simulink model "untitled"  (R2012b)
settings: Solver=ode3  StartTime=0.0  StopTime=3.5  FixedStep=1e-5/2  RelTol=1e-6
libraries: simulink x3
settings Model: Creator=Juliano  LastModifiedBy=Juliano

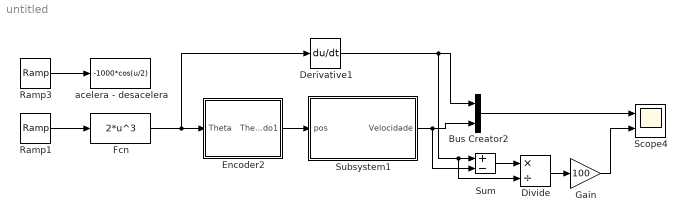
== system untitled ==
  Bus Creator2 : BusCreator  Inputs=2
  Derivative1 : Derivative
  Divide : Product  Inputs=*/
  Encoder2 : Subsystem  mask{Nr=300}
      mask prompts: Nr "Número de pulsos por revolução"
  Fcn : Fcn  Expr=2*u^3
  Gain : Gain  Gain=100
  Ramp1 : simulink/Sources/Ramp  slope=10  start=0  X0=0
  Ramp3 : simulink/Sources/Ramp  slope=2*pi  start=0  X0=0
  Scope4 : Scope  NumInputPorts=2
      settings: TickLabels=on  YMin=0~-30  YMax=30~30  SaveName=ScopeData4
  Subsystem1 : Subsystem  mask{Ts=0.01}
      mask prompts: Ts "Sampling time"
  Sum : Sum  Inputs=+-
  acelera - desacelera : Fcn  Expr=-1000*cos(u/2)
  wires:
  Ramp1/1 -> Fcn/1
  Fcn/1 -> Derivative1/1, Encoder2/1(Theta)
  Bus Creator2/1 -> Scope4/1
  Encoder2/1(Theta_amostrado1) -> Subsystem1/1(pos)
  Subsystem1/1(Velocidade) -> Sum/2, Bus Creator2/2
  Derivative1/1 -> Divide/2, Sum/1, Bus Creator2/1
  Sum/1 -> Divide/1
  Divide/1 -> Gain/1
  Gain/1 -> Scope4/2
  Ramp3/1 -> acelera - desacelera/1

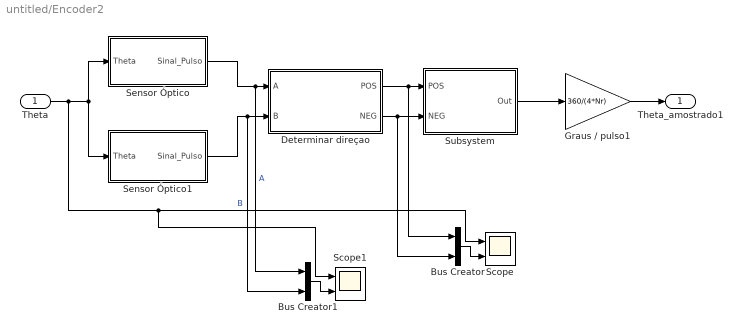
== system untitled/Encoder2 ==
  Theta : Inport
  Bus Creator : BusCreator  Inputs=2
  Bus Creator1 : BusCreator  Inputs=2
  Determinar direçao : Subsystem
  Graus / pulso1 : Gain  Gain=360/(4*Nr)  OutDataTypeStr=double
  Scope : Scope  NumInputPorts=2
      settings: YMin=-1~-5  YMax=1.5~5  SaveName=ScopeData5
  Scope1 : Scope  NumInputPorts=2
      settings: YMin=-1~-5  YMax=1.5~5  SaveName=ScopeData6
  Sensor Óptico : Subsystem
  Sensor Óptico1 : Subsystem
  Subsystem : Subsystem
  Theta_amostrado1 : Outport
  wires:
  Sensor Óptico/1(Sinal_Pulso) -> Bus Creator1/1, Determinar direçao/1(A)  "A"
  Sensor Óptico1/1(Sinal_Pulso) -> Bus Creator1/2, Determinar direçao/2(B)  "B"
  Determinar direçao/1(POS) -> Bus Creator/1, Subsystem/1(POS)
  Determinar direçao/2(NEG) -> Bus Creator/2, Subsystem/2(NEG)
  Subsystem/1(Out) -> Graus / pulso1/1
  Graus / pulso1/1 -> Theta_amostrado1/1
  Bus Creator/1 -> Scope/2
  Theta/1 -> Scope1/1, Scope/1, Sensor Óptico1/1(Theta), Sensor Óptico/1(Theta)
  Bus Creator1/1 -> Scope1/2

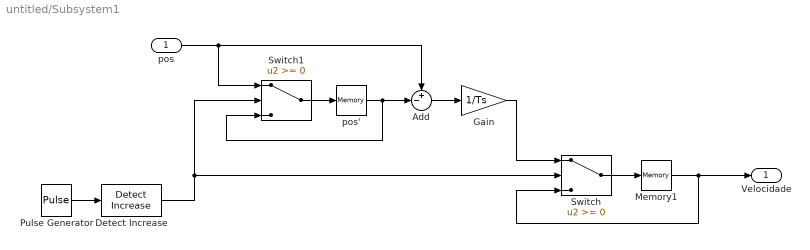
== system untitled/Subsystem1 ==
  pos : Inport
  Add : Sum  Inputs=+-|
  Detect Increase : simulink/Logic and Bit Operations/Detect Increase  vinit=0.0  InputProcessing=Inherited  OutDataTypeStr=boolean
  Gain : Gain  Gain=1/Ts
  Memory1 : Memory
  Pulse Generator : DiscretePulseGenerator  PulseType=Time based  Period=Ts  PulseWidth=50
  Switch : Switch
  Switch1 : Switch
  pos' : Memory
  Velocidade : Outport
  wires:
  pos'/1 -> Add/2, Switch1/3
  Pulse Generator/1 -> Detect Increase/1
  Add/1 -> Gain/1
  Switch1/1 -> pos'/1
  Switch/1 -> Memory1/1
  Memory1/1 -> Velocidade/1, Switch/3
  pos/1 -> Switch1/1, Add/1
  Gain/1 -> Switch/1
  Detect Increase/1 -> Switch/2, Switch1/2

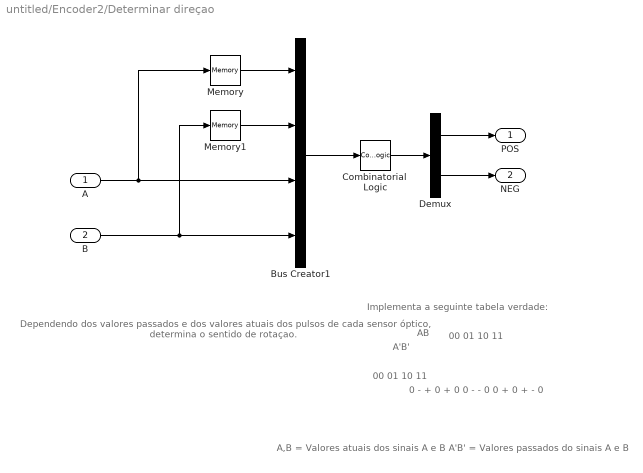
== system untitled/Encoder2/Determinar direçao ==
  note: A,B = Valores atuais dos sinais A e B
      | A'B' = Valores passados do sinais A e B
  note: A'B'
  note: AB
  note: Implementa a seguinte tabela verdade:
  note: 0	-	+	0
      | +	0	0	-
      | -	0	0	+
      | 0	+	-	0
  note: 00 01 10 11
  note: 00
      | 01
      | 10
      | 11
  note: Dependendo dos valores passados e dos valores atuais
      | dos pulsos de cada sensor óptico, determina o sentido
      | de rotaçao.
  A : Inport
  B : Inport  Port=2
  Bus Creator1 : BusCreator
  Combinatorial  Logic : CombinatorialLogic  TruthTable=[ 0 0 ; 0 1 ; 1 0 ; 0 0 ; 1 0 ; 0 0 ; 0 0 ; 0 1 ; 0 1 ; 0 0 ; 0 0 ; 1 0 ; 0 0 ; 1 0 ; 0 1 ; 0 0]
  Demux : Demux  Outputs=2
  Memory : Memory
  Memory1 : Memory
  POS : Outport
  NEG : Outport  Port=2
  wires:
  Demux/1 -> POS/1
  A/1 -> Memory/1, Bus Creator1/3
  Demux/2 -> NEG/1
  Combinatorial  Logic/1 -> Demux/1
  Memory/1 -> Bus Creator1/1
  Bus Creator1/1 -> Combinatorial  Logic/1
  Memory1/1 -> Bus Creator1/2
  B/1 -> Memory1/1, Bus Creator1/4

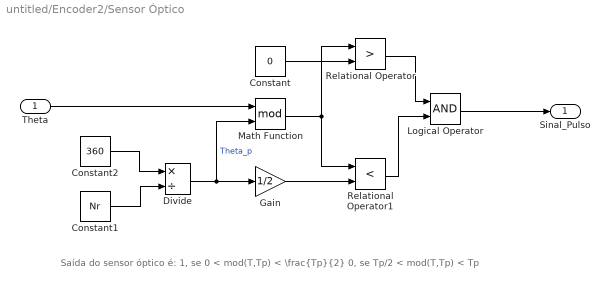
== system untitled/Encoder2/Sensor Óptico ==
  note: Saída do sensor óptico é:
      | 1, se	0 < mod(T,Tp) < \frac{Tp}{2}
      |  0, se      Tp/2 < mod(T,Tp) < Tp
  Theta : Inport
  Constant : Constant  Value=0
  Constant1 : Constant  Value=Nr
  Constant2 : Constant  Value=360
  Divide : Product  Inputs=*/
  Gain : Gain  Gain=1/2
  Logical Operator : Logic  AllPortsSameDT=off  OutDataTypeStr=boolean
  Math Function : Math  Operator=mod  SaturateOnIntegerOverflow=on
  Relational Operator : RelationalOperator  Operator=>  OutDataTypeStr=boolean
  Relational Operator1 : RelationalOperator  Operator=<  OutDataTypeStr=boolean
  Sinal_Pulso : Outport
  wires:
  Math Function/1 -> Relational Operator1/1, Relational Operator/1
  Theta/1 -> Math Function/1
  Relational Operator/1 -> Logical Operator/1
  Relational Operator1/1 -> Logical Operator/2
  Constant/1 -> Relational Operator/2
  Divide/1 -> Math Function/2, Gain/1  "Theta_p"
  Gain/1 -> Relational Operator1/2
  Logical Operator/1 -> Sinal_Pulso/1
  Constant2/1 -> Divide/1
  Constant1/1 -> Divide/2

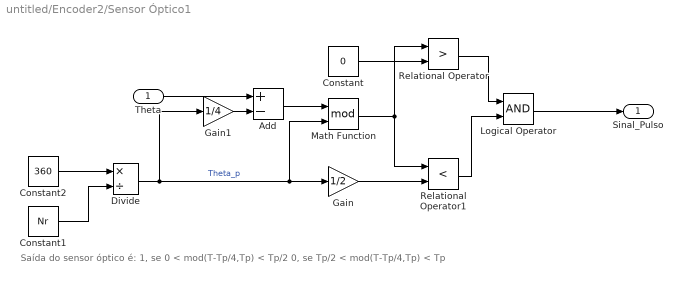
== system untitled/Encoder2/Sensor Óptico1 ==
  note: Saída do sensor óptico é:
      | 1, se	0 < mod(T-Tp/4,Tp) < Tp/2
      |  0, se     Tp/2 < mod(T-Tp/4,Tp) < Tp
  Theta : Inport
  Add : Sum  Inputs=+-
  Constant : Constant  Value=0
  Constant1 : Constant  Value=Nr
  Constant2 : Constant  Value=360
  Divide : Product  Inputs=*/
  Gain : Gain  Gain=1/2
  Gain1 : Gain  Gain=1/4
  Logical Operator : Logic  AllPortsSameDT=off  OutDataTypeStr=boolean
  Math Function : Math  Operator=mod  SaturateOnIntegerOverflow=on
  Relational Operator : RelationalOperator  Operator=>  OutDataTypeStr=boolean
  Relational Operator1 : RelationalOperator  Operator=<  OutDataTypeStr=boolean
  Sinal_Pulso : Outport
  wires:
  Constant1/1 -> Divide/2
  Constant2/1 -> Divide/1
  Logical Operator/1 -> Sinal_Pulso/1
  Gain/1 -> Relational Operator1/2
  Divide/1 -> Gain1/1, Gain/1, Math Function/2  "Theta_p"
  Constant/1 -> Relational Operator/2
  Relational Operator1/1 -> Logical Operator/2
  Relational Operator/1 -> Logical Operator/1
  Math Function/1 -> Relational Operator/1, Relational Operator1/1
  Add/1 -> Math Function/1
  Theta/1 -> Add/1
  Gain1/1 -> Add/2

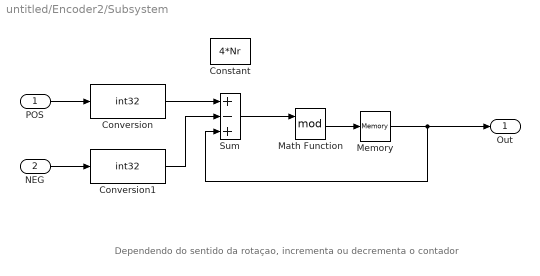
== system untitled/Encoder2/Subsystem ==
  note: Dependendo do sentido da rotaçao, incrementa ou decrementa o contador
  POS : Inport
  NEG : Inport  Port=2
  Constant : Constant  Value=4*Nr
  Conversion : DataTypeConversion  OutDataTypeStr=int32
  Conversion1 : DataTypeConversion  OutDataTypeStr=int32
  Math Function : Math  Operator=mod  SaturateOnIntegerOverflow=on
  Memory : Memory
  Sum : Sum  Inputs=+-+
  Out : Outport
  wires:
  Sum/1 -> Math Function/1
  Memory/1 -> Out/1, Sum/3
  Math Function/1 -> Memory/1
  POS/1 -> Conversion/1
  Conversion/1 -> Sum/1
  Conversion1/1 -> Sum/2
  NEG/1 -> Conversion1/1
